simulink library "srx_platform"  (Simulink 8.2)
settings: Solver=ode1  StartTime=0.0  StopTime=Inf  FixedStep=0.001  RelTol=1e-3
PostLoadFcn:
  | , if any(exist('dsrtsu_mdlpostloadfcn', 'file') == [2, 3, 6]), try dsrtsu_mdlpostloadfcn('Execute', bdroot); catch fprintf('Error in PostLoadFcn (dsrtsu_mdlpostloadfcn) for model "%s":\n %s\n', bdroot, lasterr); end, end,
libraries: rtican x23, rtiethernetudplib x4, srx_initialize x4, rtiflashlib x2, topr5_adapter x1
(part 4 of 6)

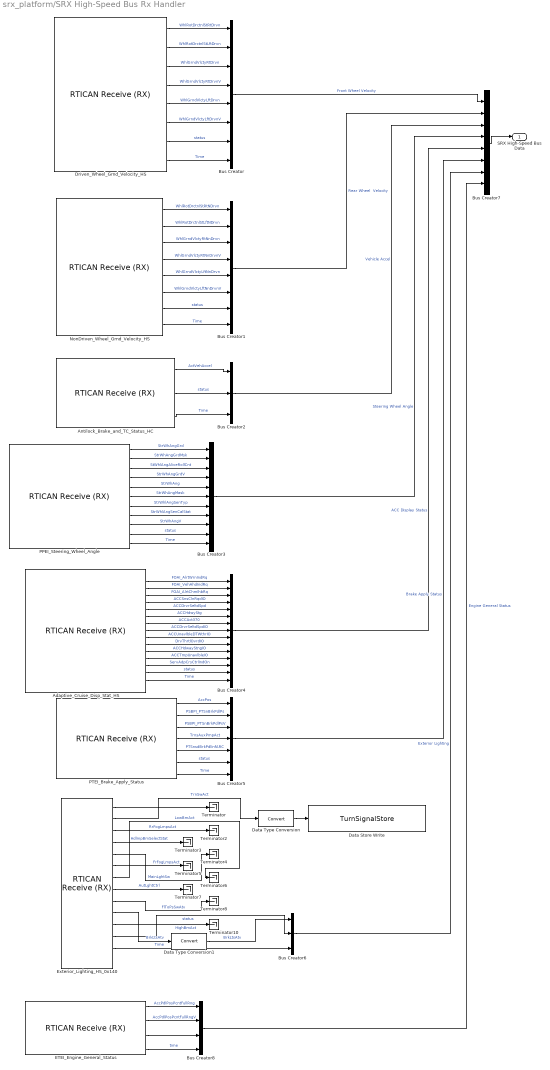
== system srx_platform/SRX High-Speed Bus Rx Handler ==
  Adaptive_Cruise_Disp_Stat_HS : rtican/RTICAN Receive (RX)   Reserved1=[]  Reserved2=[]  Reserved3=[]  Reserved4=[]  SfcnMessage=[]  Msg_Struct=[]  BoardTypeNo=[]  BoardNo=[]  ChannelNo=[]  Parameters=[]  DialogFcn=[]  UnitName=[]  Revision=[]  UnitValues=[]  DSProperties=struct('RTI',struct('Version',uint32(5),'BlockType',struct('isSLSource',uint8(1),'isSLSink',uint8(1),'isHWSource',uint8(0),'isHWSink',uint8(0),'isSetup',uint8(0),'isInline',uint8(1),'isNonInline',uint8(0),'isInterrupt',uint8(0),'isChannelwise',uint8(0)),'IOBoardType','RTICAN','UnitType','MESSAGE','Identifier','RX','DialogType','MSVC','BlockSet','RTICAN','SlaveProcessor','CAN'))  RTIBlockInterface=struct('OutputPortsWidth',int32([1 1 1 1 1 1 1 1 1 1 1 1 1 1 1]),'OutputPortsActive',[1 1 1 1 1 1 1 1 1 1 1 1 1 1 1],'OutputPortsName',{{'FOAI_AlrtWrnIndRq','FOAI_VehAhdIndRq','FOAI_AlrtChmIhbRq','ACCSnsClnRqdIO','ACCDrvrSeltdSpd','ACCHdwyStg','ACCAct370','ACCDrvrSeltdSpdIO','ACCUnavlbleDTWthrIO','DrvThrtlOvrdIO','ACCHdwayStngIO','ACCTmpUnavlbleIO','ServAdpCrsCtrlIndOn',['RX status'],['RX time']}},'OutputPortsDataType',{{'SS_UINT8','SS_UINT8','SS_BOOLEAN','SS_UINT32','SS_DOUBLE','SS_UINT8','SS_BOOLEAN','SS_BOOLEAN','SS_BOOLEAN','SS_BOOLEAN','SS_BOOLEAN','SS_BOOLEAN','SS_BOOLEAN','SS_DOUBLE','SS_DOUBLE'}},'OutputPortsLabel',{{'FOAI_AlrtWrnIndRq','FOAI_VehAhdIndRq','FOAI_AlrtChmIhbRq','ACCSnsClnRqdIO','ACCDrvrSeltdSpd','ACCHdwyStg','ACCAct370','ACCDrvrSeltdSpdIO','ACCUnavlbleDTWthrIO','DrvThrtlOvrdIO','ACCHdwayStngIO','ACCTmpUnavlbleIO','ServAdpCrsCtrlIndOn','',''}},'OutputPortsLabelMode','ON','InputPortsWidth',int32(0),'InputPortsActive',0,'DialogFcn','rtican_message_interface_gui','BlockDisplay',{{'','center'}},'IconTransparency','on','ParameterTunableNames',{{}},'InitLevel',3,'BlockName',struct('Token',{{'Adaptive_Cruise_Disp_Stat_HS'}}),'SampleTime',{{-1}},'TriggerPort',{{'none'}},'EnablePort',{{'none'}})  RTIBlockParameters=struct('BoardTypeNo',{{1,'OFF',[]}},'BoardNo',{{1,'ON',[1 16]}},'ChannelNo',{{1,'ON',[1 2]}},'Parameters',{{struct('DataFileSupport',struct('DataFileSelectedMaster',1,'DataFileSelectedLocal',1,'DataFileName','c:\users\leidos\development\carmaplatform\microautobox\src\data_files\srx_high_speed.dbc|','DataFileDate',{{{['12-Aug-2015 17:10:44']}}},'SelectedFile','..\data_files\srx_high_speed.dbc','InterfaceFcn','rtican_dbc_file_parser'),'Options',struct('StatusSelected',1,'TimeSelected',1,'DeltaTimeSelected',0,'BytePortSelected',0,'MessageLengthSelected',0,'TriggerPort',struct('Selected',0,'TriggerType',0),'UserCoding',struct('Selected',0,'InterfaceFile','UserDecodingFile','FcnName','UserDecodeFcn','InportSelected',0,'InportWidth',1,'OutportSelected',0,'OutportWidth',1),'EnablePortSelected',0,'SignalOnPortnameSelected',1,'UseRXService',1),'Message',struct('MsgOnBlocknameSelected',1,'MsgName','Adaptive_Cruise_Disp_Stat_HS','MsgIdFormat',0,'MsgId',880,'MsgLength',6,'NumSignals',13,'SampleTime',-1,'Signal',struct('SgnName',{'FOAI_AlrtWrnIndRq','FOAI_VehAhdIndRq','FOAI_AlrtChmIhbRq','ACCSnsClnRqdIO','ACCDrvrSeltdSpd','ACCHdwyStg','ACCAct370','ACCDrvrSeltdSpdIO','ACCUnavlbleDTWthrIO','DrvThrtlOvrdIO','ACCHdwayStngIO','ACCTmpUnavlbleIO','ServAdpCrsCtrlIndOn'},'SgnStartBit',{0,4,8,14,16,28,31,41,42,43,44,45,47},'SgnLength',{4,4,1,32,12,3,1,1,1,1,1,1,1},'SgnType',{0,0,0,0,0,0,0,0,0,0,0,0,0},'ModeValue',{-1,-1,-1,-1,-1,-1,-1,-1,-1,-1,-1,-1,-1},'DataType',{0,0,0,0,0,0,0,0,0,0,0,0,0},'ByteLayout',{2,2,2,2,2,2,2,2,2,2,2,2,2},'Factor',{1,1,1,1,0.0625,1,1,1,1,1,1,1,1},'Offset',{0,0,0,0,0,0,0,0,0,0,0,0,0},'SgnComment',{{['Forward Object Alert Indications : Alert Warning Indication Request']},{['Forward Object Alert Indications : Vehicle Ahead Indication Request']},{['Forward Object Alert Indications : Alert Warning Chime Inhibit Request']},{['Adaptive Cruise Control Sensor Cleaning Required Indication On']},{''},{['Adaptive Cruise Control Headway Setting']},{['Adaptive Cruise Control Active']},{['Adaptive Cruise Control Driver Selected Speed Indication On']},{['Adaptive Cruise Unavailable Due To Weather Indication On']},{['Driver Throttle Override Indication On']},{['Adaptive Cruise Control Headway Setting Indication On']},{['Adaptive Cruise Control Temporarily Unavailable Indication On']},{['Service Adaptive Cruise Control Indication On']}},'SgnUnit',{'','','','','km/h','','','','','','','',''},'Min',{0,0,0,0,0,0,0,0,0,0,0,0,0},'Max',{0,0,0,0,0,0,0,0,0,0,0,0,0},'SLDataType',{'SS_UINT8','SS_UINT8','SS_BOOLEAN','SS_UINT32','SS_DOUBLE','SS_UINT8','SS_BOOLEAN','SS_BOOLEAN','SS_BOOLEAN','SS_BOOLEAN','SS_BOOLEAN','SS_BOOLEAN','SS_BOOLEAN'}),'MsgIdNumFormat',0,'MsgComment',{{''}}),'Version',1.2,'general',struct('isFromLib',0)),'OFF',[]}},'GroupId',{{struct('Group',{{'RTICAN'}},'No',1,'Behavior',{{'NAMECHANGE'}},'BlockType',{{'SINK'}},'NameChangeFlag',0),'OFF',[]}},'SFcnRTICANMessage',{{struct('MsgType','RX','SFcnPortType','Scalar','MsgName','Adaptive_Cruise_Disp_Stat_HS','MsgIdFormat','STD','MsgId',880,'MsgLength',6,'NumSignals',13,'SampleTime',-1,'Signal',struct('SgnName',{'FOAI_AlrtWrnIndRq','FOAI_VehAhdIndRq','FOAI_AlrtChmIhbRq','ACCSnsClnRqdIO','ACCDrvrSeltdSpd','ACCHdwyStg','ACCAct370','ACCDrvrSeltdSpdIO','ACCUnavlbleDTWthrIO','DrvThrtlOvrdIO','ACCHdwayStngIO','ACCTmpUnavlbleIO','ServAdpCrsCtrlIndOn'},'SgnStartBit',{0,4,8,14,16,28,31,41,42,43,44,45,47},'SgnLength',{4,4,1,32,12,3,1,1,1,1,1,1,1},'SgnType',{'standard','standard','standard','standard','standard','standard','standard','standard','standard','standard','standard','standard','standard'},'ModeValue',{-1,-1,-1,-1,-1,-1,-1,-1,-1,-1,-1,-1,-1},'DataType',{['unsigned int'],['unsigned int'],['unsigned int'],['unsigned int'],['unsigned int'],['unsigned int'],['unsigned int'],['unsigned int'],['unsigned int'],['unsigned int'],['unsigned int'],['unsigned int'],['unsigned int']},'ByteLayout',{['motorola back.'],['motorola back.'],['motorola back.'],['motorola back.'],['motorola back.'],['motorola back.'],['motorola back.'],['motorola back.'],['motorola back.'],['motorola back.'],['motorola back.'],['motorola back.'],['motorola back.']},'Factor',{1,1,1,1,0.0625,1,1,1,1,1,1,1,1},'Offset',{0,0,0,0,0,0,0,0,0,0,0,0,0},'SLDataType',{'SS_UINT8','SS_UINT8','SS_BOOLEAN','SS_UINT32','SS_DOUBLE','SS_UINT8','SS_BOOLEAN','SS_BOOLEAN','SS_BOOLEAN','SS_BOOLEAN','SS_BOOLEAN','SS_BOOLEAN','SS_BOOLEAN'}),'StatusSelected','yes','TimeSelected','yes','DeltaTimeSelected','no','BytePortSelected','no','MessageLengthSelected','no','TriggerPort',struct('Selected','no','TriggerType',0),'UserCoding',struct('Selected','no','InterfaceFile','UserDecodingFile','FcnName','UserDecodeFcn','InportSelected','no','InportWidth',1,'OutportSelected','no','OutportWidth',1),'EnablePortSelected','no','UseRXService','yes','BoardType','DS1','BoardNo',1,'ControllerNo',1),'OFF',[]}},'TLCFileName',{{'rtican_rx_message','OFF',[]}})  RTISFcnParameters=struct('SFcnRTICANMessage','struct','TLCFileName','char')  RTIBlockParaDefault=struct('BoardTypeNo',4302,'BoardNo',1,'ChannelNo',1,'Parameters',struct('DataFileSupport',struct('DataFileSelectedMaster',0,'DataFileSelectedLocal',0,'DataFileName','','DataFileDate','','SelectedFile',['<no file selected>']),'Options',struct('StatusSelected',1,'TimeSelected',1,'DeltaTimeSelected',1,'BytePortSelected',0,'MessageLengthSelected',0,'TriggerPort',struct('Selected',0,'TriggerType','rising'),'UserCoding',struct('Selected',0,'InterfaceFile','UserDecodingFile','FcnName','UserDecodeFcn','InportSelected',0,'InportWidth',1,'OutportSelected',0,'OutportWidth',1),'EnablePortSelected',0,'SignalOnPortnameSelected',1,'UseRXService',0),'Message',struct('MsgOnBlocknameSelected',0,'MsgName',['RX Message'],'MsgIdFormat',0,'MsgId',100,'MsgLength',8,'NumSignals',1,'SampleTime',-1,'Signal',struct('SgnName',['RX signal'],'SgnStartBit',0,'SgnLength',8,'SgnType',0,'ModeValue',-1,'DataType',0,'SLDataType','SS_DOUBLE','ByteLayout',0,'Factor',1,'Offset',0,'Min',0,'Max',255,'SgnComment',{{}},'SgnUnit',''),'MsgIdNumFormat',0,'MsgComment',{{''}}),'Version',1.2,'general',struct('isFromLib',1)),'GroupId',struct('Group',{{'RTICAN'}},'No',1,'Behavior',{{'NAMECHANGE'}},'BlockType',{{'SINK'}},'NameChangeFlag',0),'SFcnRTICANMessage',struct('MsgType','RX','MsgName',['RX Message'],'MsgIdFormat','STD','MsgId',100,'MsgLength',8,'NumSignals',1,'SampleTime',-1,'Signal',struct('SgnName',['RX signal'],'SgnStartBit',0,'SgnLength',8,'SgnType','standard','ModeValue',-1,'DataType',['unsigned int'],'ByteLayout',['little endian'],'SLDataType','SS_DOUBLE','Factor',1,'Offset',0),'StatusSelected','yes','TimeSelected','yes','DeltaTimeSelected','yes','BytePortSelected','no','MessageLengthSelected','no','EnablePortSelected','no','UserCoding',struct('Selected','no','InterfaceFile','UserDecodingFile','FcnName','UserDecodeFcn','InportSelected','no','InportWidth',1,'OutportSelected','no','OutportWidth',1),'TriggerPort',struct('Selected','no','TriggerType','rising'),'UseRXService','no','BoardType','DS4302','BoardNo',1,'ControllerNo',1,'SFcnPortType','Scalar'),'TLCFileName','rtican_rx_message')
      settings: AttributesFormatString=Group Id: RTICAN1\n
  Antilock_Brake_and_TC_Status_HC : rtican/RTICAN Receive (RX)   Reserved1=[]  Reserved2=[]  Reserved3=[]  Reserved4=[]  SfcnMessage=[]  Msg_Struct=[]  BoardTypeNo=[]  BoardNo=[]  ChannelNo=[]  Parameters=[]  DialogFcn=[]  UnitName=[]  Revision=[]  UnitValues=[]  DSProperties=struct('RTI',struct('Version',uint32(5),'BlockType',struct('isSLSource',uint8(1),'isSLSink',uint8(1),'isHWSource',uint8(0),'isHWSink',uint8(0),'isSetup',uint8(0),'isInline',uint8(1),'isNonInline',uint8(0),'isInterrupt',uint8(0),'isChannelwise',uint8(0)),'IOBoardType','RTICAN','UnitType','MESSAGE','Identifier','RX','DialogType','MSVC','BlockSet','RTICAN','SlaveProcessor','CAN'))  RTIBlockInterface=struct('OutputPortsWidth',int32([1 1 1]),'OutputPortsActive',[1 1 1],'OutputPortsName',{{'ActVehAccel',['RX status'],['RX time']}},'OutputPortsDataType',{{'SS_DOUBLE','SS_DOUBLE','SS_DOUBLE'}},'OutputPortsLabel',{{'ActVehAccel','',''}},'OutputPortsLabelMode','ON','InputPortsWidth',int32(0),'InputPortsActive',0,'DialogFcn','rtican_message_interface_gui','BlockDisplay',{{'','center'}},'IconTransparency','on','ParameterTunableNames',{{}},'InitLevel',3,'BlockName',struct('Token',{{'Antilock_Brake_and_TC_Status_HC'}}),'SampleTime',{{-1}},'TriggerPort',{{'none'}},'EnablePort',{{'none'}})  RTIBlockParameters=struct('BoardTypeNo',{{1,'OFF',[]}},'BoardNo',{{1,'ON',[1 16]}},'ChannelNo',{{1,'ON',[1 2]}},'Parameters',{{struct('DataFileSupport',struct('DataFileSelectedMaster',1,'DataFileSelectedLocal',1,'DataFileName','c:\users\leidos\development\carmaplatform\microautobox\src\data_files\srx_high_speed.dbc|','DataFileDate',{{{['12-Aug-2015 17:10:44']}}},'SelectedFile','..\data_files\srx_high_speed.dbc'),'Options',struct('StatusSelected',1,'TimeSelected',1,'DeltaTimeSelected',0,'BytePortSelected',0,'MessageLengthSelected',0,'TriggerPort',struct('Selected',0,'TriggerType',0),'UserCoding',struct('Selected',0,'InterfaceFile','UserDecodingFile','FcnName','UserDecodeFcn','InportSelected',0,'InportWidth',1,'OutportSelected',0,'OutportWidth',1),'EnablePortSelected',0,'SignalOnPortnameSelected',1,'UseRXService',1),'Message',struct('MsgOnBlocknameSelected',1,'MsgName','Antilock_Brake_and_TC_Status_HC','MsgIdFormat',0,'MsgId',381,'MsgLength',6,'NumSignals',1,'SampleTime',-1,'Signal',struct('SgnName','ActVehAccel','SgnStartBit',0,'SgnLength',12,'SgnType',0,'ModeValue',-1,'DataType',1,'ByteLayout',2,'Factor',0.01,'Offset',0,'SgnComment',{{''}},'SgnUnit','m/s^2','Min',0,'Max',0,'SLDataType','SS_DOUBLE'),'MsgIdNumFormat',0,'MsgComment',{{''}}),'Version',1.2,'general',struct('isFromLib',0)),'OFF',[]}},'GroupId',{{struct('Group',{{'RTICAN'}},'No',1,'Behavior',{{'NAMECHANGE'}},'BlockType',{{'SINK'}},'NameChangeFlag',0),'OFF',[]}},'SFcnRTICANMessage',{{struct('MsgType','RX','SFcnPortType','Scalar','MsgName','Antilock_Brake_and_TC_Status_HC','MsgIdFormat','STD','MsgId',381,'MsgLength',6,'NumSignals',1,'SampleTime',-1,'Signal',struct('SgnName','ActVehAccel','SgnStartBit',0,'SgnLength',12,'SgnType','standard','ModeValue',-1,'DataType',['signed int'],'ByteLayout',['motorola back.'],'Factor',0.01,'Offset',0,'SLDataType','SS_DOUBLE'),'StatusSelected','yes','TimeSelected','yes','DeltaTimeSelected','no','BytePortSelected','no','MessageLengthSelected','no','TriggerPort',struct('Selected','no','TriggerType',0),'UserCoding',struct('Selected','no','InterfaceFile','UserDecodingFile','FcnName','UserDecodeFcn','InportSelected','no','InportWidth',1,'OutportSelected','no','OutportWidth',1),'EnablePortSelected','no','UseRXService','yes','BoardType','DS1','BoardNo',1,'ControllerNo',1),'OFF',[]}},'TLCFileName',{{'rtican_rx_message','OFF',[]}})  RTISFcnParameters=struct('SFcnRTICANMessage','struct','TLCFileName','char')  RTIBlockParaDefault=struct('BoardTypeNo',4302,'BoardNo',1,'ChannelNo',1,'Parameters',struct('DataFileSupport',struct('DataFileSelectedMaster',0,'DataFileSelectedLocal',0,'DataFileName','','DataFileDate','','SelectedFile',['<no file selected>']),'Options',struct('StatusSelected',1,'TimeSelected',1,'DeltaTimeSelected',1,'BytePortSelected',0,'MessageLengthSelected',0,'TriggerPort',struct('Selected',0,'TriggerType','rising'),'UserCoding',struct('Selected',0,'InterfaceFile','UserDecodingFile','FcnName','UserDecodeFcn','InportSelected',0,'InportWidth',1,'OutportSelected',0,'OutportWidth',1),'EnablePortSelected',0,'SignalOnPortnameSelected',1,'UseRXService',0),'Message',struct('MsgOnBlocknameSelected',0,'MsgName',['RX Message'],'MsgIdFormat',0,'MsgId',100,'MsgLength',8,'NumSignals',1,'SampleTime',-1,'Signal',struct('SgnName',['RX signal'],'SgnStartBit',0,'SgnLength',8,'SgnType',0,'ModeValue',-1,'DataType',0,'SLDataType','SS_DOUBLE','ByteLayout',0,'Factor',1,'Offset',0,'Min',0,'Max',255,'SgnComment',{{}},'SgnUnit',''),'MsgIdNumFormat',0,'MsgComment',{{''}}),'Version',1.2,'general',struct('isFromLib',1)),'GroupId',struct('Group',{{'RTICAN'}},'No',1,'Behavior',{{'NAMECHANGE'}},'BlockType',{{'SINK'}},'NameChangeFlag',0),'SFcnRTICANMessage',struct('MsgType','RX','MsgName',['RX Message'],'MsgIdFormat','STD','MsgId',100,'MsgLength',8,'NumSignals',1,'SampleTime',-1,'Signal',struct('SgnName',['RX signal'],'SgnStartBit',0,'SgnLength',8,'SgnType','standard','ModeValue',-1,'DataType',['unsigned int'],'ByteLayout',['little endian'],'SLDataType','SS_DOUBLE','Factor',1,'Offset',0),'StatusSelected','yes','TimeSelected','yes','DeltaTimeSelected','yes','BytePortSelected','no','MessageLengthSelected','no','EnablePortSelected','no','UserCoding',struct('Selected','no','InterfaceFile','UserDecodingFile','FcnName','UserDecodeFcn','InportSelected','no','InportWidth',1,'OutportSelected','no','OutportWidth',1),'TriggerPort',struct('Selected','no','TriggerType','rising'),'UseRXService','no','BoardType','DS4302','BoardNo',1,'ControllerNo',1,'SFcnPortType','Scalar'),'TLCFileName','rtican_rx_message')
      settings: AttributesFormatString=Group Id: RTICAN1\n
  Bus Creator : BusCreator  Inputs=8  NonVirtualBus=on
  Bus Creator1 : BusCreator  Inputs=8
  Bus Creator2 : BusCreator  Inputs=3
  Bus Creator3 : BusCreator  Inputs=11
  Bus Creator4 : BusCreator  Inputs=15
  Bus Creator5 : BusCreator  Inputs=7
  Bus Creator6 : BusCreator  Inputs=3
  Bus Creator7 : BusCreator  Inputs=8
  Bus Creator8 : BusCreator
  Data Store Write : DataStoreWrite  DataStoreName=TurnSignalStore
  Data Type Conversion : DataTypeConversion
  Data Type Conversion1 : DataTypeConversion
  Driven_Wheel_Grnd_Velocity_HS : rtican/RTICAN Receive (RX)   Reserved1=[]  Reserved2=[]  Reserved3=[]  Reserved4=[]  SfcnMessage=[]  Msg_Struct=[]  BoardTypeNo=[]  BoardNo=[]  ChannelNo=[]  Parameters=[]  DialogFcn=[]  UnitName=[]  Revision=[]  UnitValues=[]  DSProperties=struct('RTI',struct('Version',uint32(5),'BlockType',struct('isSLSource',uint8(1),'isSLSink',uint8(1),'isHWSource',uint8(0),'isHWSink',uint8(0),'isSetup',uint8(0),'isInline',uint8(1),'isNonInline',uint8(0),'isInterrupt',uint8(0),'isChannelwise',uint8(0)),'IOBoardType','RTICAN','UnitType','MESSAGE','Identifier','RX','DialogType','MSVC','BlockSet','RTICAN','SlaveProcessor','CAN'))  RTIBlockInterface=struct('OutputPortsWidth',int32([1 1 1 1 1 1 1 1]),'OutputPortsActive',[1 1 1 1 1 1 1 1],'OutputPortsName',{{'WhlRotDrctnlStRtDrvn','WhlRotDrctnlStLftDrvn','WhlGrndVlctyRtDrvn','WhlGrndVlctyRtDrvnV','WhlGrndVlctyLftDrvn','WhlGrndVlctyLftDrvnV',['RX status'],['RX time']}},'OutputPortsDataType',{{'SS_UINT8','SS_UINT8','SS_DOUBLE','SS_BOOLEAN','SS_DOUBLE','SS_BOOLEAN','SS_DOUBLE','SS_DOUBLE'}},'OutputPortsLabel',{{'WhlRotDrctnlStRtDrvn','WhlRotDrctnlStLftDrvn','WhlGrndVlctyRtDrvn','WhlGrndVlctyRtDrvnV','WhlGrndVlctyLftDrvn','WhlGrndVlctyLftDrvnV','',''}},'OutputPortsLabelMode','ON','InputPortsWidth',int32(0),'InputPortsActive',0,'DialogFcn','rtican_message_interface_gui','BlockDisplay',{{'','center'}},'IconTransparency','on','ParameterTunableNames',{{}},'InitLevel',3,'BlockName',struct('Token',{{'Driven_Wheel_Grnd_Velocity_HS'}}),'SampleTime',{{-1}},'TriggerPort',{{'none'}},'EnablePort',{{'none'}})  RTIBlockParameters=struct('BoardTypeNo',{{1,'OFF',[]}},'BoardNo',{{1,'ON',[1 16]}},'ChannelNo',{{1,'ON',[1 2]}},'Parameters',{{struct('DataFileSupport',struct('DataFileSelectedMaster',1,'DataFileSelectedLocal',1,'DataFileName','c:\users\leidos\development\carmaplatform\microautobox\src\data_files\srx_high_speed.dbc|','DataFileDate',{{{['12-Aug-2015 17:10:44']}}},'SelectedFile','..\data_files\srx_high_speed.dbc','InterfaceFcn','rtican_dbc_file_parser'),'Options',struct('StatusSelected',1,'TimeSelected',1,'DeltaTimeSelected',0,'BytePortSelected',0,'MessageLengthSelected',0,'TriggerPort',struct('Selected',0,'TriggerType',0),'UserCoding',struct('Selected',0,'InterfaceFile','UserDecodingFile','FcnName','UserDecodeFcn','InportSelected',0,'InportWidth',1,'OutportSelected',0,'OutportWidth',1),'EnablePortSelected',0,'SignalOnPortnameSelected',1,'UseRXService',1),'Message',struct('MsgOnBlocknameSelected',1,'MsgName','Driven_Wheel_Grnd_Velocity_HS','MsgIdFormat',0,'MsgId',840,'MsgLength',5,'NumSignals',6,'SampleTime',-1,'Signal',struct('SgnName',{'WhlRotDrctnlStRtDrvn','WhlRotDrctnlStLftDrvn','WhlGrndVlctyRtDrvn','WhlGrndVlctyRtDrvnV','WhlGrndVlctyLftDrvn','WhlGrndVlctyLftDrvnV'},'SgnStartBit',{0,3,8,22,24,38},'SgnLength',{3,3,14,1,14,1},'SgnType',{0,0,0,0,0,0},'ModeValue',{-1,-1,-1,-1,-1,-1},'DataType',{0,0,0,0,0,0},'ByteLayout',{2,2,2,2,2,2},'Factor',{1,1,0.03125,1,0.03125,1},'Offset',{0,0,0,0,0,0},'SgnComment',{{''},{''},{''},{''},{''},{''}},'SgnUnit',{'','','km/h','','km/h',''},'Min',{0,0,0,0,0,0},'Max',{0,0,0,0,0,0},'SLDataType',{'SS_UINT8','SS_UINT8','SS_DOUBLE','SS_BOOLEAN','SS_DOUBLE','SS_BOOLEAN'}),'MsgIdNumFormat',0,'MsgComment',{{''}}),'Version',1.2,'general',struct('isFromLib',0)),'OFF',[]}},'GroupId',{{struct('Group',{{'RTICAN'}},'No',1,'Behavior',{{'NAMECHANGE'}},'BlockType',{{'SINK'}},'NameChangeFlag',0),'OFF',[]}},'SFcnRTICANMessage',{{struct('MsgType','RX','SFcnPortType','Scalar','MsgName','Driven_Wheel_Grnd_Velocity_HS','MsgIdFormat','STD','MsgId',840,'MsgLength',5,'NumSignals',6,'SampleTime',-1,'Signal',struct('SgnName',{'WhlRotDrctnlStRtDrvn','WhlRotDrctnlStLftDrvn','WhlGrndVlctyRtDrvn','WhlGrndVlctyRtDrvnV','WhlGrndVlctyLftDrvn','WhlGrndVlctyLftDrvnV'},'SgnStartBit',{0,3,8,22,24,38},'SgnLength',{3,3,14,1,14,1},'SgnType',{'standard','standard','standard','standard','standard','standard'},'ModeValue',{-1,-1,-1,-1,-1,-1},'DataType',{['unsigned int'],['unsigned int'],['unsigned int'],['unsigned int'],['unsigned int'],['unsigned int']},'ByteLayout',{['motorola back.'],['motorola back.'],['motorola back.'],['motorola back.'],['motorola back.'],['motorola back.']},'Factor',{1,1,0.03125,1,0.03125,1},'Offset',{0,0,0,0,0,0},'SLDataType',{'SS_UINT8','SS_UINT8','SS_DOUBLE','SS_BOOLEAN','SS_DOUBLE','SS_BOOLEAN'}),'StatusSelected','yes','TimeSelected','yes','DeltaTimeSelected','no','BytePortSelected','no','MessageLengthSelected','no','TriggerPort',struct('Selected','no','TriggerType',0),'UserCoding',struct('Selected','no','InterfaceFile','UserDecodingFile','FcnName','UserDecodeFcn','InportSelected','no','InportWidth',1,'OutportSelected','no','OutportWidth',1),'EnablePortSelected','no','UseRXService','yes','BoardType','DS1','BoardNo',1,'ControllerNo',1),'OFF',[]}},'TLCFileName',{{'rtican_rx_message','OFF',[]}})  RTISFcnParameters=struct('SFcnRTICANMessage','struct','TLCFileName','char')  RTIBlockParaDefault=struct('BoardTypeNo',4302,'BoardNo',1,'ChannelNo',1,'Parameters',struct('DataFileSupport',struct('DataFileSelectedMaster',0,'DataFileSelectedLocal',0,'DataFileName','','DataFileDate','','SelectedFile',['<no file selected>']),'Options',struct('StatusSelected',1,'TimeSelected',1,'DeltaTimeSelected',1,'BytePortSelected',0,'MessageLengthSelected',0,'TriggerPort',struct('Selected',0,'TriggerType','rising'),'UserCoding',struct('Selected',0,'InterfaceFile','UserDecodingFile','FcnName','UserDecodeFcn','InportSelected',0,'InportWidth',1,'OutportSelected',0,'OutportWidth',1),'EnablePortSelected',0,'SignalOnPortnameSelected',1,'UseRXService',0),'Message',struct('MsgOnBlocknameSelected',0,'MsgName',['RX Message'],'MsgIdFormat',0,'MsgId',100,'MsgLength',8,'NumSignals',1,'SampleTime',-1,'Signal',struct('SgnName',['RX signal'],'SgnStartBit',0,'SgnLength',8,'SgnType',0,'ModeValue',-1,'DataType',0,'SLDataType','SS_DOUBLE','ByteLayout',0,'Factor',1,'Offset',0,'Min',0,'Max',255,'SgnComment',{{}},'SgnUnit',''),'MsgIdNumFormat',0,'MsgComment',{{''}}),'Version',1.2,'general',struct('isFromLib',1)),'GroupId',struct('Group',{{'RTICAN'}},'No',1,'Behavior',{{'NAMECHANGE'}},'BlockType',{{'SINK'}},'NameChangeFlag',0),'SFcnRTICANMessage',struct('MsgType','RX','MsgName',['RX Message'],'MsgIdFormat','STD','MsgId',100,'MsgLength',8,'NumSignals',1,'SampleTime',-1,'Signal',struct('SgnName',['RX signal'],'SgnStartBit',0,'SgnLength',8,'SgnType','standard','ModeValue',-1,'DataType',['unsigned int'],'ByteLayout',['little endian'],'SLDataType','SS_DOUBLE','Factor',1,'Offset',0),'StatusSelected','yes','TimeSelected','yes','DeltaTimeSelected','yes','BytePortSelected','no','MessageLengthSelected','no','EnablePortSelected','no','UserCoding',struct('Selected','no','InterfaceFile','UserDecodingFile','FcnName','UserDecodeFcn','InportSelected','no','InportWidth',1,'OutportSelected','no','OutportWidth',1),'TriggerPort',struct('Selected','no','TriggerType','rising'),'UseRXService','no','BoardType','DS4302','BoardNo',1,'ControllerNo',1,'SFcnPortType','Scalar'),'TLCFileName','rtican_rx_message')
      settings: AttributesFormatString=Group Id: RTICAN1\n
  ETEI_Engine_General_Status : rtican/RTICAN Receive (RX)   Reserved1=[]  Reserved2=[]  Reserved3=[]  Reserved4=[]  SfcnMessage=[]  Msg_Struct=[]  BoardTypeNo=[]  BoardNo=[]  ChannelNo=[]  Parameters=[]  DialogFcn=[]  UnitName=[]  Revision=[]  UnitValues=[]  DSProperties=struct('RTI',struct('Version',uint32(5),'BlockType',struct('isSLSource',uint8(1),'isSLSink',uint8(1),'isHWSource',uint8(0),'isHWSink',uint8(0),'isSetup',uint8(0),'isInline',uint8(1),'isNonInline',uint8(0),'isInterrupt',uint8(0),'isChannelwise',uint8(0)),'IOBoardType','RTICAN','UnitType','MESSAGE','Identifier','RX','DialogType','MSVC','BlockSet','RTICAN','SlaveProcessor','CAN'))  RTIBlockInterface=struct('OutputPortsWidth',int32([1 1 1 1]),'OutputPortsActive',[1 1 1 1],'OutputPortsName',{{'AccPdlPosPcntFullRng','AccPdlPosPcntFullRngV',['RX status'],['RX time']}},'OutputPortsDataType',{{'SS_DOUBLE','SS_BOOLEAN','SS_DOUBLE','SS_DOUBLE'}},'OutputPortsLabel',{{'AccPdlPosPcntFullRng','AccPdlPosPcntFullRngV','',''}},'OutputPortsLabelMode','ON','InputPortsWidth',int32(0),'InputPortsActive',0,'DialogFcn','rtican_message_interface_gui','BlockDisplay',{{'','center'}},'IconTransparency','on','ParameterTunableNames',{{}},'InitLevel',3,'BlockName',struct('Token',{{'ETEI_Engine_General_Status'}}),'SampleTime',{{-1}},'TriggerPort',{{'none'}},'EnablePort',{{'none'}})  RTIBlockParameters=struct('BoardTypeNo',{{1,'OFF',[]}},'BoardNo',{{1,'ON',[1 16]}},'ChannelNo',{{1,'ON',[1 2]}},'Parameters',{{struct('DataFileSupport',struct('DataFileSelectedMaster',1,'DataFileSelectedLocal',1,'DataFileName','c:\users\leidos\development\carmaplatform\microautobox\src\data_files\srx_high_speed.dbc|','DataFileDate',{{{['21-Aug-2015 11:37:23']}}},'SelectedFile','..\data_files\srx_high_speed.dbc'),'Options',struct('StatusSelected',1,'TimeSelected',1,'DeltaTimeSelected',0,'BytePortSelected',0,'MessageLengthSelected',0,'TriggerPort',struct('Selected',0,'TriggerType',0),'UserCoding',struct('Selected',0,'InterfaceFile','UserDecodingFile','FcnName','UserDecodeFcn','InportSelected',0,'InportWidth',1,'OutportSelected',0,'OutportWidth',1),'EnablePortSelected',0,'SignalOnPortnameSelected',1,'UseRXService',0),'Message',struct('MsgOnBlocknameSelected',1,'MsgName','ETEI_Engine_General_Status','MsgIdFormat',0,'MsgId',417,'MsgLength',8,'NumSignals',2,'SampleTime',-1,'Signal',struct('SgnName',{'AccPdlPosPcntFullRng','AccPdlPosPcntFullRngV'},'SgnStartBit',{8,41},'SgnLength',{8,1},'SgnType',{0,0},'ModeValue',{-1,-1},'DataType',{0,0},'ByteLayout',{2,2},'Factor',{0.392157,1},'Offset',{0,0},'SgnComment',{{''},{''}},'SgnUnit',{'%',''},'Min',{0,0},'Max',{0,0},'SLDataType',{'SS_DOUBLE','SS_BOOLEAN'}),'MsgIdNumFormat',0,'MsgComment',{{''}}),'Version',1.2,'general',struct('isFromLib',0)),'OFF',[]}},'GroupId',{{struct('Group',{{'RTICAN'}},'No',1,'Behavior',{{'NAMECHANGE'}},'BlockType',{{'SINK'}},'NameChangeFlag',0),'OFF',[]}},'SFcnRTICANMessage',{{struct('MsgType','RX','SFcnPortType','Scalar','MsgName','ETEI_Engine_General_Status','MsgIdFormat','STD','MsgId',417,'MsgLength',8,'NumSignals',2,'SampleTime',-1,'Signal',struct('SgnName',{'AccPdlPosPcntFullRng','AccPdlPosPcntFullRngV'},'SgnStartBit',{8,41},'SgnLength',{8,1},'SgnType',{'standard','standard'},'ModeValue',{-1,-1},'DataType',{['unsigned int'],['unsigned int']},'ByteLayout',{['motorola back.'],['motorola back.']},'Factor',{0.392157,1},'Offset',{0,0},'SLDataType',{'SS_DOUBLE','SS_BOOLEAN'}),'StatusSelected','yes','TimeSelected','yes','DeltaTimeSelected','no','BytePortSelected','no','MessageLengthSelected','no','TriggerPort',struct('Selected','no','TriggerType',0),'UserCoding',struct('Selected','no','InterfaceFile','UserDecodingFile','FcnName','UserDecodeFcn','InportSelected','no','InportWidth',1,'OutportSelected','no','OutportWidth',1),'EnablePortSelected','no','UseRXService','no','BoardType','DS1','BoardNo',1,'ControllerNo',1),'OFF',[]}},'TLCFileName',{{'rtican_rx_message','OFF',[]}})  RTISFcnParameters=struct('SFcnRTICANMessage','struct','TLCFileName','char')  RTIBlockParaDefault=struct('BoardTypeNo',4302,'BoardNo',1,'ChannelNo',1,'Parameters',struct('DataFileSupport',struct('DataFileSelectedMaster',0,'DataFileSelectedLocal',0,'DataFileName','','DataFileDate','','SelectedFile',['<no file selected>']),'Options',struct('StatusSelected',1,'TimeSelected',1,'DeltaTimeSelected',1,'BytePortSelected',0,'MessageLengthSelected',0,'TriggerPort',struct('Selected',0,'TriggerType','rising'),'UserCoding',struct('Selected',0,'InterfaceFile','UserDecodingFile','FcnName','UserDecodeFcn','InportSelected',0,'InportWidth',1,'OutportSelected',0,'OutportWidth',1),'EnablePortSelected',0,'SignalOnPortnameSelected',1,'UseRXService',0),'Message',struct('MsgOnBlocknameSelected',0,'MsgName',['RX Message'],'MsgIdFormat',0,'MsgId',100,'MsgLength',8,'NumSignals',1,'SampleTime',-1,'Signal',struct('SgnName',['RX signal'],'SgnStartBit',0,'SgnLength',8,'SgnType',0,'ModeValue',-1,'DataType',0,'SLDataType','SS_DOUBLE','ByteLayout',0,'Factor',1,'Offset',0,'Min',0,'Max',255,'SgnComment',{{}},'SgnUnit',''),'MsgIdNumFormat',0,'MsgComment',{{''}}),'Version',1.2,'general',struct('isFromLib',1)),'GroupId',struct('Group',{{'RTICAN'}},'No',1,'Behavior',{{'NAMECHANGE'}},'BlockType',{{'SINK'}},'NameChangeFlag',0),'SFcnRTICANMessage',struct('MsgType','RX','MsgName',['RX Message'],'MsgIdFormat','STD','MsgId',100,'MsgLength',8,'NumSignals',1,'SampleTime',-1,'Signal',struct('SgnName',['RX signal'],'SgnStartBit',0,'SgnLength',8,'SgnType','standard','ModeValue',-1,'DataType',['unsigned int'],'ByteLayout',['little endian'],'SLDataType','SS_DOUBLE','Factor',1,'Offset',0),'StatusSelected','yes','TimeSelected','yes','DeltaTimeSelected','yes','BytePortSelected','no','MessageLengthSelected','no','EnablePortSelected','no','UserCoding',struct('Selected','no','InterfaceFile','UserDecodingFile','FcnName','UserDecodeFcn','InportSelected','no','InportWidth',1,'OutportSelected','no','OutportWidth',1),'TriggerPort',struct('Selected','no','TriggerType','rising'),'UseRXService','no','BoardType','DS4302','BoardNo',1,'ControllerNo',1,'SFcnPortType','Scalar'),'TLCFileName','rtican_rx_message')
      settings: AttributesFormatString=Group Id: RTICAN1\n
  Exterior_Lighting_HS_0x140 : rtican/RTICAN Receive (RX)   Reserved1=[]  Reserved2=[]  Reserved3=[]  Reserved4=[]  SfcnMessage=[]  Msg_Struct=[]  BoardTypeNo=[]  BoardNo=[]  ChannelNo=[]  Parameters=[]  DialogFcn=[]  UnitName=[]  Revision=[]  UnitValues=[]  DSProperties=struct('RTI',struct('Version',uint32(5),'BlockType',struct('isSLSource',uint8(1),'isSLSink',uint8(1),'isHWSource',uint8(0),'isHWSink',uint8(0),'isSetup',uint8(0),'isInline',uint8(1),'isNonInline',uint8(0),'isInterrupt',uint8(0),'isChannelwise',uint8(0)),'IOBoardType','RTICAN','UnitType','MESSAGE','Identifier','RX','DialogType','MSVC','BlockSet','RTICAN','SlaveProcessor','CAN'))  RTIBlockInterface=struct('OutputPortsWidth',int32([1 1 1 1 1 1 1 1 1 1 1 1 1 1]),'OutputPortsActive',[1 1 1 1 1 1 1 1 1 1 1 1 1 1],'OutputPortsName',{{'OtsdAmbtLtLvlStat','TrnSwAct','RrFogLmpsAct','HdlmpBmSelectStat','MainLghtSw','FrFogLmpsAct','LowBmAct','AutLghtCtrl','FlToPsSwAtv','BrkLtsAtv','HighBmAct',['RX status'],['RX time'],['RX delta time']}},'OutputPortsDataType',{{'SS_DOUBLE','SS_DOUBLE','SS_DOUBLE','SS_DOUBLE','SS_DOUBLE','SS_DOUBLE','SS_DOUBLE','SS_DOUBLE','SS_DOUBLE','SS_DOUBLE','SS_DOUBLE','SS_DOUBLE','SS_DOUBLE','SS_DOUBLE'}},'OutputPortsLabel',{{'OtsdAmbtLtLvlStat','TrnSwAct','RrFogLmpsAct','HdlmpBmSelectStat','MainLghtSw','FrFogLmpsAct','LowBmAct','AutLghtCtrl','FlToPsSwAtv','BrkLtsAtv','HighBmAct','','',''}},'OutputPortsLabelMode','ON','InputPortsWidth',int32(0),'InputPortsActive',0,'DialogFcn','rtican_message_interface_gui','BlockDisplay',{{'','center'}},'IconTransparency','on','ParameterTunableNames',{{}},'InitLevel',3,'BlockName',struct('Token',{{'Exterior_Lighting_HS_0x140'}}),'SampleTime',{{-1}},'TriggerPort',{{'none'}},'EnablePort',{{'none'}})  RTIBlockParameters=struct('BoardTypeNo',{{1,'OFF',[]}},'BoardNo',{{1,'ON',[1 16]}},'ChannelNo',{{1,'ON',[1 2]}},'Parameters',{{struct('DataFileSupport',struct('DataFileSelectedMaster',0,'DataFileSelectedLocal',0,'DataFileName',['<no datafile support>|'],'DataFileDate','','SelectedFile',['<no file selected>']),'Options',struct('StatusSelected',1,'TimeSelected',1,'DeltaTimeSelected',1,'BytePortSelected',0,'MessageLengthSelected',0,'TriggerPort',struct('Selected',0,'TriggerType',0),'UserCoding',struct('Selected',0,'InterfaceFile','UserDecodingFile','FcnName','UserDecodeFcn','InportSelected',0,'InportWidth',1,'OutportSelected',0,'OutportWidth',1),'EnablePortSelected',0,'SignalOnPortnameSelected',1,'UseRXService',1),'Message',struct('MsgOnBlocknameSelected',1,'MsgName','Exterior_Lighting_HS_0x140','MsgIdFormat',0,'MsgId',320,'MsgLength',3,'NumSignals',11,'SampleTime',-1,'Signal',struct('SgnName',{'OtsdAmbtLtLvlStat','TrnSwAct','RrFogLmpsAct','HdlmpBmSelectStat','MainLghtSw','FrFogLmpsAct','LowBmAct','AutLghtCtrl','FlToPsSwAtv','BrkLtsAtv','HighBmAct'},'SgnStartBit',{0,2,8,8,11,16,17,20,21,22,23},'SgnLength',{2,2,1,2,2,1,1,1,1,1,1},'SgnType',{0,0,0,0,0,0,0,0,0,0,0},'ModeValue',{-1,-1,-1,-1,-1,-1,-1,-1,-1,-1,-1},'DataType',{0,0,0,0,0,0,0,0,0,0,0},'ByteLayout',{2,2,2,2,2,2,2,2,2,2,2},'Factor',{1,1,1,1,1,1,1,1,1,1,1},'Offset',{0,0,0,0,0,0,0,0,0,0,0},'SgnComment',{{''},{''},{''},{''},{''},{''},{''},{''},{''},{''},{''}},'SgnUnit',{'','','','','','','','','','',''},'Min',{0,0,0,0,0,0,0,0,0,0,0},'Max',{255,255,255,255,255,255,255,255,255,255,255},'SLDataType',{'SS_DOUBLE','SS_DOUBLE','SS_DOUBLE','SS_DOUBLE','SS_DOUBLE','SS_DOUBLE','SS_DOUBLE','SS_DOUBLE','SS_DOUBLE','SS_DOUBLE','SS_DOUBLE'}),'MsgIdNumFormat',1,'MsgComment',{{''}}),'Version',1.2,'general',struct('isFromLib',0)),'OFF',[]}},'GroupId',{{struct('Group',{{'RTICAN'}},'No',1,'Behavior',{{'NAMECHANGE'}},'BlockType',{{'SINK'}},'NameChangeFlag',0),'OFF',[]}},'SFcnRTICANMessage',{{struct('MsgType','RX','SFcnPortType','Scalar','MsgName','Exterior_Lighting_HS_0x140','MsgIdFormat','STD','MsgId',320,'MsgLength',3,'NumSignals',11,'SampleTime',-1,'Signal',struct('SgnName',{'OtsdAmbtLtLvlStat','TrnSwAct','RrFogLmpsAct','HdlmpBmSelectStat','MainLghtSw','FrFogLmpsAct','LowBmAct','AutLghtCtrl','FlToPsSwAtv','BrkLtsAtv','HighBmAct'},'SgnStartBit',{0,2,8,8,11,16,17,20,21,22,23},'SgnLength',{2,2,1,2,2,1,1,1,1,1,1},'SgnType',{'standard','standard','standard','standard','standard','standard','standard','standard','standard','standard','standard'},'ModeValue',{-1,-1,-1,-1,-1,-1,-1,-1,-1,-1,-1},'DataType',{['unsigned int'],['unsigned int'],['unsigned int'],['unsigned int'],['unsigned int'],['unsigned int'],['unsigned int'],['unsigned int'],['unsigned int'],['unsigned int'],['unsigned int']},'ByteLayout',{['motorola back.'],['motorola back.'],['motorola back.'],['motorola back.'],['motorola back.'],['motorola back.'],['motorola back.'],['motorola back.'],['motorola back.'],['motorola back.'],['motorola back.']},'Factor',{1,1,1,1,1,1,1,1,1,1,1},'Offset',{0,0,0,0,0,0,0,0,0,0,0},'SLDataType',{'SS_DOUBLE','SS_DOUBLE','SS_DOUBLE','SS_DOUBLE','SS_DOUBLE','SS_DOUBLE','SS_DOUBLE','SS_DOUBLE','SS_DOUBLE','SS_DOUBLE','SS_DOUBLE'}),'StatusSelected','yes','TimeSelected','yes','DeltaTimeSelected','yes','BytePortSelected','no','MessageLengthSelected','no','TriggerPort',struct('Selected','no','TriggerType',0),'UserCoding',struct('Selected','no','InterfaceFile','UserDecodingFile','FcnName','UserDecodeFcn','InportSelected','no','InportWidth',1,'OutportSelected','no','OutportWidth',1),'EnablePortSelected','no','UseRXService','yes','BoardType','DS1','BoardNo',1,'ControllerNo',1),'OFF',[]}},'TLCFileName',{{'rtican_rx_message','OFF',[]}})  RTISFcnParameters=struct('SFcnRTICANMessage','struct','TLCFileName','char')  RTIBlockParaDefault=struct('BoardTypeNo',4302,'BoardNo',1,'ChannelNo',1,'Parameters',struct('DataFileSupport',struct('DataFileSelectedMaster',0,'DataFileSelectedLocal',0,'DataFileName','','DataFileDate','','SelectedFile',['<no file selected>']),'Options',struct('StatusSelected',1,'TimeSelected',1,'DeltaTimeSelected',1,'BytePortSelected',0,'MessageLengthSelected',0,'TriggerPort',struct('Selected',0,'TriggerType','rising'),'UserCoding',struct('Selected',0,'InterfaceFile','UserDecodingFile','FcnName','UserDecodeFcn','InportSelected',0,'InportWidth',1,'OutportSelected',0,'OutportWidth',1),'EnablePortSelected',0,'SignalOnPortnameSelected',1,'UseRXService',0),'Message',struct('MsgOnBlocknameSelected',0,'MsgName',['RX Message'],'MsgIdFormat',0,'MsgId',100,'MsgLength',8,'NumSignals',1,'SampleTime',-1,'Signal',struct('SgnName',['RX signal'],'SgnStartBit',0,'SgnLength',8,'SgnType',0,'ModeValue',-1,'DataType',0,'SLDataType','SS_DOUBLE','ByteLayout',0,'Factor',1,'Offset',0,'Min',0,'Max',255,'SgnComment',{{}},'SgnUnit',''),'MsgIdNumFormat',0,'MsgComment',{{''}}),'Version',1.2,'general',struct('isFromLib',1)),'GroupId',struct('Group',{{'RTICAN'}},'No',1,'Behavior',{{'NAMECHANGE'}},'BlockType',{{'SINK'}},'NameChangeFlag',0),'SFcnRTICANMessage',struct('MsgType','RX','MsgName',['RX Message'],'MsgIdFormat','STD','MsgId',100,'MsgLength',8,'NumSignals',1,'SampleTime',-1,'Signal',struct('SgnName',['RX signal'],'SgnStartBit',0,'SgnLength',8,'SgnType','standard','ModeValue',-1,'DataType',['unsigned int'],'ByteLayout',['little endian'],'SLDataType','SS_DOUBLE','Factor',1,'Offset',0),'StatusSelected','yes','TimeSelected','yes','DeltaTimeSelected','yes','BytePortSelected','no','MessageLengthSelected','no','EnablePortSelected','no','UserCoding',struct('Selected','no','InterfaceFile','UserDecodingFile','FcnName','UserDecodeFcn','InportSelected','no','InportWidth',1,'OutportSelected','no','OutportWidth',1),'TriggerPort',struct('Selected','no','TriggerType','rising'),'UseRXService','no','BoardType','DS4302','BoardNo',1,'ControllerNo',1,'SFcnPortType','Scalar'),'TLCFileName','rtican_rx_message')
      settings: AttributesFormatString=Group Id: RTICAN1\n
  NonDriven_Wheel_Grnd_Velocity_HS : rtican/RTICAN Receive (RX)   Reserved1=[]  Reserved2=[]  Reserved3=[]  Reserved4=[]  SfcnMessage=[]  Msg_Struct=[]  BoardTypeNo=[]  BoardNo=[]  ChannelNo=[]  Parameters=[]  DialogFcn=[]  UnitName=[]  Revision=[]  UnitValues=[]  DSProperties=struct('RTI',struct('Version',uint32(5),'BlockType',struct('isSLSource',uint8(1),'isSLSink',uint8(1),'isHWSource',uint8(0),'isHWSink',uint8(0),'isSetup',uint8(0),'isInline',uint8(1),'isNonInline',uint8(0),'isInterrupt',uint8(0),'isChannelwise',uint8(0)),'IOBoardType','RTICAN','UnitType','MESSAGE','Identifier','RX','DialogType','MSVC','BlockSet','RTICAN','SlaveProcessor','CAN'))  RTIBlockInterface=struct('OutputPortsWidth',int32([1 1 1 1 1 1 1 1]),'OutputPortsActive',[1 1 1 1 1 1 1 1],'OutputPortsName',{{'WhlRotDrctnlStRtNDrvn','WhlRotDrctnlStLftNDrvn','WhlGrndVlctyRtNnDrvn','WhlGrndVlctyRtNnDrvnV','WhlGrndVlctyLftNnDrvn','WhlGrndVlctyLftNnDrvnV',['RX status'],['RX time']}},'OutputPortsDataType',{{'SS_UINT8','SS_UINT8','SS_DOUBLE','SS_BOOLEAN','SS_DOUBLE','SS_BOOLEAN','SS_DOUBLE','SS_DOUBLE'}},'OutputPortsLabel',{{'WhlRotDrctnlStRtNDrvn','WhlRotDrctnlStLftNDrvn','WhlGrndVlctyRtNnDrvn','WhlGrndVlctyRtNnDrvnV','WhlGrndVlctyLftNnDrvn','WhlGrndVlctyLftNnDrvnV','',''}},'OutputPortsLabelMode','ON','InputPortsWidth',int32(0),'InputPortsActive',0,'DialogFcn','rtican_message_interface_gui','BlockDisplay',{{'','center'}},'IconTransparency','on','ParameterTunableNames',{{}},'InitLevel',3,'BlockName',struct('Token',{{'NonDriven_Wheel_Grnd_Velocity_HS'}}),'SampleTime',{{-1}},'TriggerPort',{{'none'}},'EnablePort',{{'none'}})  RTIBlockParameters=struct('BoardTypeNo',{{1,'OFF',[]}},'BoardNo',{{1,'ON',[1 16]}},'ChannelNo',{{1,'ON',[1 2]}},'Parameters',{{struct('DataFileSupport',struct('DataFileSelectedMaster',1,'DataFileSelectedLocal',1,'DataFileName','c:\users\leidos\development\carmaplatform\microautobox\src\data_files\srx_high_speed.dbc|','DataFileDate',{{{['12-Aug-2015 17:10:44']}}},'SelectedFile','..\data_files\srx_high_speed.dbc','InterfaceFcn','rtican_dbc_file_parser'),'Options',struct('StatusSelected',1,'TimeSelected',1,'DeltaTimeSelected',0,'BytePortSelected',0,'MessageLengthSelected',0,'TriggerPort',struct('Selected',0,'TriggerType',0),'UserCoding',struct('Selected',0,'InterfaceFile','UserDecodingFile','FcnName','UserDecodeFcn','InportSelected',0,'InportWidth',1,'OutportSelected',0,'OutportWidth',1),'EnablePortSelected',0,'SignalOnPortnameSelected',1,'UseRXService',1),'Message',struct('MsgOnBlocknameSelected',1,'MsgName','NonDriven_Wheel_Grnd_Velocity_HS','MsgIdFormat',0,'MsgId',842,'MsgLength',5,'NumSignals',6,'SampleTime',-1,'Signal',struct('SgnName',{'WhlRotDrctnlStRtNDrvn','WhlRotDrctnlStLftNDrvn','WhlGrndVlctyRtNnDrvn','WhlGrndVlctyRtNnDrvnV','WhlGrndVlctyLftNnDrvn','WhlGrndVlctyLftNnDrvnV'},'SgnStartBit',{0,3,8,22,24,38},'SgnLength',{3,3,14,1,14,1},'SgnType',{0,0,0,0,0,0},'ModeValue',{-1,-1,-1,-1,-1,-1},'DataType',{0,0,0,0,0,0},'ByteLayout',{2,2,2,2,2,2},'Factor',{1,1,0.03125,1,0.03125,1},'Offset',{0,0,0,0,0,0},'SgnComment',{{''},{''},{''},{''},{''},{''}},'SgnUnit',{'','','km/h','','km/h',''},'Min',{0,0,0,0,0,0},'Max',{0,0,0,0,0,0},'SLDataType',{'SS_UINT8','SS_UINT8','SS_DOUBLE','SS_BOOLEAN','SS_DOUBLE','SS_BOOLEAN'}),'MsgIdNumFormat',0,'MsgComment',{{''}}),'Version',1.2,'general',struct('isFromLib',0)),'OFF',[]}},'GroupId',{{struct('Group',{{'RTICAN'}},'No',1,'Behavior',{{'NAMECHANGE'}},'BlockType',{{'SINK'}},'NameChangeFlag',0),'OFF',[]}},'SFcnRTICANMessage',{{struct('MsgType','RX','SFcnPortType','Scalar','MsgName','NonDriven_Wheel_Grnd_Velocity_HS','MsgIdFormat','STD','MsgId',842,'MsgLength',5,'NumSignals',6,'SampleTime',-1,'Signal',struct('SgnName',{'WhlRotDrctnlStRtNDrvn','WhlRotDrctnlStLftNDrvn','WhlGrndVlctyRtNnDrvn','WhlGrndVlctyRtNnDrvnV','WhlGrndVlctyLftNnDrvn','WhlGrndVlctyLftNnDrvnV'},'SgnStartBit',{0,3,8,22,24,38},'SgnLength',{3,3,14,1,14,1},'SgnType',{'standard','standard','standard','standard','standard','standard'},'ModeValue',{-1,-1,-1,-1,-1,-1},'DataType',{['unsigned int'],['unsigned int'],['unsigned int'],['unsigned int'],['unsigned int'],['unsigned int']},'ByteLayout',{['motorola back.'],['motorola back.'],['motorola back.'],['motorola back.'],['motorola back.'],['motorola back.']},'Factor',{1,1,0.03125,1,0.03125,1},'Offset',{0,0,0,0,0,0},'SLDataType',{'SS_UINT8','SS_UINT8','SS_DOUBLE','SS_BOOLEAN','SS_DOUBLE','SS_BOOLEAN'}),'StatusSelected','yes','TimeSelected','yes','DeltaTimeSelected','no','BytePortSelected','no','MessageLengthSelected','no','TriggerPort',struct('Selected','no','TriggerType',0),'UserCoding',struct('Selected','no','InterfaceFile','UserDecodingFile','FcnName','UserDecodeFcn','InportSelected','no','InportWidth',1,'OutportSelected','no','OutportWidth',1),'EnablePortSelected','no','UseRXService','yes','BoardType','DS1','BoardNo',1,'ControllerNo',1),'OFF',[]}},'TLCFileName',{{'rtican_rx_message','OFF',[]}})  RTISFcnParameters=struct('SFcnRTICANMessage','struct','TLCFileName','char')  RTIBlockParaDefault=struct('BoardTypeNo',4302,'BoardNo',1,'ChannelNo',1,'Parameters',struct('DataFileSupport',struct('DataFileSelectedMaster',0,'DataFileSelectedLocal',0,'DataFileName','','DataFileDate','','SelectedFile',['<no file selected>']),'Options',struct('StatusSelected',1,'TimeSelected',1,'DeltaTimeSelected',1,'BytePortSelected',0,'MessageLengthSelected',0,'TriggerPort',struct('Selected',0,'TriggerType','rising'),'UserCoding',struct('Selected',0,'InterfaceFile','UserDecodingFile','FcnName','UserDecodeFcn','InportSelected',0,'InportWidth',1,'OutportSelected',0,'OutportWidth',1),'EnablePortSelected',0,'SignalOnPortnameSelected',1,'UseRXService',0),'Message',struct('MsgOnBlocknameSelected',0,'MsgName',['RX Message'],'MsgIdFormat',0,'MsgId',100,'MsgLength',8,'NumSignals',1,'SampleTime',-1,'Signal',struct('SgnName',['RX signal'],'SgnStartBit',0,'SgnLength',8,'SgnType',0,'ModeValue',-1,'DataType',0,'SLDataType','SS_DOUBLE','ByteLayout',0,'Factor',1,'Offset',0,'Min',0,'Max',255,'SgnComment',{{}},'SgnUnit',''),'MsgIdNumFormat',0,'MsgComment',{{''}}),'Version',1.2,'general',struct('isFromLib',1)),'GroupId',struct('Group',{{'RTICAN'}},'No',1,'Behavior',{{'NAMECHANGE'}},'BlockType',{{'SINK'}},'NameChangeFlag',0),'SFcnRTICANMessage',struct('MsgType','RX','MsgName',['RX Message'],'MsgIdFormat','STD','MsgId',100,'MsgLength',8,'NumSignals',1,'SampleTime',-1,'Signal',struct('SgnName',['RX signal'],'SgnStartBit',0,'SgnLength',8,'SgnType','standard','ModeValue',-1,'DataType',['unsigned int'],'ByteLayout',['little endian'],'SLDataType','SS_DOUBLE','Factor',1,'Offset',0),'StatusSelected','yes','TimeSelected','yes','DeltaTimeSelected','yes','BytePortSelected','no','MessageLengthSelected','no','EnablePortSelected','no','UserCoding',struct('Selected','no','InterfaceFile','UserDecodingFile','FcnName','UserDecodeFcn','InportSelected','no','InportWidth',1,'OutportSelected','no','OutportWidth',1),'TriggerPort',struct('Selected','no','TriggerType','rising'),'UseRXService','no','BoardType','DS4302','BoardNo',1,'ControllerNo',1,'SFcnPortType','Scalar'),'TLCFileName','rtican_rx_message')
      settings: AttributesFormatString=Group Id: RTICAN1\n
  PPEI_Steering_Wheel_Angle : rtican/RTICAN Receive (RX)   Reserved1=[]  Reserved2=[]  Reserved3=[]  Reserved4=[]  SfcnMessage=[]  Msg_Struct=[]  BoardTypeNo=[]  BoardNo=[]  ChannelNo=[]  Parameters=[]  DialogFcn=[]  UnitName=[]  Revision=[]  UnitValues=[]  DSProperties=struct('RTI',struct('Version',uint32(5),'BlockType',struct('isSLSource',uint8(1),'isSLSink',uint8(1),'isHWSource',uint8(0),'isHWSink',uint8(0),'isSetup',uint8(0),'isInline',uint8(1),'isNonInline',uint8(0),'isInterrupt',uint8(0),'isChannelwise',uint8(0)),'IOBoardType','RTICAN','UnitType','MESSAGE','Identifier','RX','DialogType','MSVC','BlockSet','RTICAN','SlaveProcessor','CAN'))  RTIBlockInterface=struct('OutputPortsWidth',int32([1 1 1 1 1 1 1 1 1 1 1]),'OutputPortsActive',[1 1 1 1 1 1 1 1 1 1 1],'OutputPortsName',{{'StrWhAngGrd','StrWhAngGrdMsk','StWhlAngAliveRollCnt','StrWhAngGrdV','StrWhAng','StrWhAngMask','StrWhlAngSenTyp','StrWhlAngSenCalStat','StrWhAngV',['RX status'],['RX time']}},'OutputPortsDataType',{{'SS_INT16','SS_BOOLEAN','SS_UINT8','SS_BOOLEAN','SS_DOUBLE','SS_BOOLEAN','SS_UINT8','SS_UINT8','SS_BOOLEAN','SS_DOUBLE','SS_DOUBLE'}},'OutputPortsLabel',{{'StrWhAngGrd','StrWhAngGrdMsk','StWhlAngAliveRollCnt','StrWhAngGrdV','StrWhAng','StrWhAngMask','StrWhlAngSenTyp','StrWhlAngSenCalStat','StrWhAngV','',''}},'OutputPortsLabelMode','ON','InputPortsWidth',int32(0),'InputPortsActive',0,'DialogFcn','rtican_message_interface_gui','BlockDisplay',{{'','center'}},'IconTransparency','on','ParameterTunableNames',{{}},'InitLevel',3,'BlockName',struct('Token',{{'PPEI_Steering_Wheel_Angle'}}),'SampleTime',{{-1}},'TriggerPort',{{'none'}},'EnablePort',{{'none'}})  RTIBlockParameters=struct('BoardTypeNo',{{1,'OFF',[]}},'BoardNo',{{1,'ON',[1 16]}},'ChannelNo',{{1,'ON',[1 2]}},'Parameters',{{struct('DataFileSupport',struct('DataFileSelectedMaster',1,'DataFileSelectedLocal',1,'DataFileName','c:\users\leidos\development\carmaplatform\microautobox\src\data_files\srx_high_speed.dbc|','DataFileDate',{{{['12-Aug-2015 17:10:44']}}},'SelectedFile','..\data_files\srx_high_speed.dbc'),'Options',struct('StatusSelected',1,'TimeSelected',1,'DeltaTimeSelected',0,'BytePortSelected',0,'MessageLengthSelected',0,'TriggerPort',struct('Selected',0,'TriggerType',0),'UserCoding',struct('Selected',0,'InterfaceFile','UserDecodingFile','FcnName','UserDecodeFcn','InportSelected',0,'InportWidth',1,'OutportSelected',0,'OutportWidth',1),'EnablePortSelected',0,'SignalOnPortnameSelected',1,'UseRXService',1),'Message',struct('MsgOnBlocknameSelected',1,'MsgName','PPEI_Steering_Wheel_Angle','MsgIdFormat',0,'MsgId',485,'MsgLength',8,'NumSignals',9,'SampleTime',-1,'Signal',struct('SgnName',{'StrWhAngGrd','StrWhAngGrdMsk','StWhlAngAliveRollCnt','StrWhAngGrdV','StrWhAng','StrWhAngMask','StrWhlAngSenTyp','StrWhlAngSenCalStat','StrWhAngV'},'SgnStartBit',{24,36,37,39,40,58,59,61,63},'SgnLength',{12,1,2,1,16,1,2,2,1},'SgnType',{0,0,0,0,0,0,0,0,0},'ModeValue',{-1,-1,-1,-1,-1,-1,-1,-1,-1},'DataType',{1,0,0,0,1,0,0,0,0},'ByteLayout',{2,2,2,2,2,2,2,2,2},'Factor',{1,1,1,1,0.0625,1,1,1,1},'Offset',{0,0,0,0,0,0,0,0,0},'SgnComment',{{['Steering Wheel Angle Gradient']},{['Steering Wheel Angle Gradient Mask']},{['Steering Wheel Angle Alive Rolling Count']},{['Steering Wheel Angle Gradient Validity']},{['Steering Wheel Angle']},{''},{['Steering Wheel Angle Sensor Type']},{['Steering Wheel Angle Sensor Calibration Status']},{['Steering Wheel Angle Validity']}},'SgnUnit',{'','','','','deg','','','',''},'Min',{0,0,0,0,0,0,0,0,0},'Max',{0,0,0,0,0,0,0,0,0},'SLDataType',{'SS_INT16','SS_BOOLEAN','SS_UINT8','SS_BOOLEAN','SS_DOUBLE','SS_BOOLEAN','SS_UINT8','SS_UINT8','SS_BOOLEAN'}),'MsgIdNumFormat',0,'MsgComment',{{''}}),'Version',1.2,'general',struct('isFromLib',0)),'OFF',[]}},'GroupId',{{struct('Group',{{'RTICAN'}},'No',1,'Behavior',{{'NAMECHANGE'}},'BlockType',{{'SINK'}},'NameChangeFlag',0),'OFF',[]}},'SFcnRTICANMessage',{{struct('MsgType','RX','SFcnPortType','Scalar','MsgName','PPEI_Steering_Wheel_Angle','MsgIdFormat','STD','MsgId',485,'MsgLength',8,'NumSignals',9,'SampleTime',-1,'Signal',struct('SgnName',{'StrWhAngGrd','StrWhAngGrdMsk','StWhlAngAliveRollCnt','StrWhAngGrdV','StrWhAng','StrWhAngMask','StrWhlAngSenTyp','StrWhlAngSenCalStat','StrWhAngV'},'SgnStartBit',{24,36,37,39,40,58,59,61,63},'SgnLength',{12,1,2,1,16,1,2,2,1},'SgnType',{'standard','standard','standard','standard','standard','standard','standard','standard','standard'},'ModeValue',{-1,-1,-1,-1,-1,-1,-1,-1,-1},'DataType',{['signed int'],['unsigned int'],['unsigned int'],['unsigned int'],['signed int'],['unsigned int'],['unsigned int'],['unsigned int'],['unsigned int']},'ByteLayout',{['motorola back.'],['motorola back.'],['motorola back.'],['motorola back.'],['motorola back.'],['motorola back.'],['motorola back.'],['motorola back.'],['motorola back.']},'Factor',{1,1,1,1,0.0625,1,1,1,1},'Offset',{0,0,0,0,0,0,0,0,0},'SLDataType',{'SS_INT16','SS_BOOLEAN','SS_UINT8','SS_BOOLEAN','SS_DOUBLE','SS_BOOLEAN','SS_UINT8','SS_UINT8','SS_BOOLEAN'}),'StatusSelected','yes','TimeSelected','yes','DeltaTimeSelected','no','BytePortSelected','no','MessageLengthSelected','no','TriggerPort',struct('Selected','no','TriggerType',0),'UserCoding',struct('Selected','no','InterfaceFile','UserDecodingFile','FcnName','UserDecodeFcn','InportSelected','no','InportWidth',1,'OutportSelected','no','OutportWidth',1),'EnablePortSelected','no','UseRXService','yes','BoardType','DS1','BoardNo',1,'ControllerNo',1),'OFF',[]}},'TLCFileName',{{'rtican_rx_message','OFF',[]}})  RTISFcnParameters=struct('SFcnRTICANMessage','struct','TLCFileName','char')  RTIBlockParaDefault=struct('BoardTypeNo',4302,'BoardNo',1,'ChannelNo',1,'Parameters',struct('DataFileSupport',struct('DataFileSelectedMaster',0,'DataFileSelectedLocal',0,'DataFileName','','DataFileDate','','SelectedFile',['<no file selected>']),'Options',struct('StatusSelected',1,'TimeSelected',1,'DeltaTimeSelected',1,'BytePortSelected',0,'MessageLengthSelected',0,'TriggerPort',struct('Selected',0,'TriggerType','rising'),'UserCoding',struct('Selected',0,'InterfaceFile','UserDecodingFile','FcnName','UserDecodeFcn','InportSelected',0,'InportWidth',1,'OutportSelected',0,'OutportWidth',1),'EnablePortSelected',0,'SignalOnPortnameSelected',1,'UseRXService',0),'Message',struct('MsgOnBlocknameSelected',0,'MsgName',['RX Message'],'MsgIdFormat',0,'MsgId',100,'MsgLength',8,'NumSignals',1,'SampleTime',-1,'Signal',struct('SgnName',['RX signal'],'SgnStartBit',0,'SgnLength',8,'SgnType',0,'ModeValue',-1,'DataType',0,'SLDataType','SS_DOUBLE','ByteLayout',0,'Factor',1,'Offset',0,'Min',0,'Max',255,'SgnComment',{{}},'SgnUnit',''),'MsgIdNumFormat',0,'MsgComment',{{''}}),'Version',1.2,'general',struct('isFromLib',1)),'GroupId',struct('Group',{{'RTICAN'}},'No',1,'Behavior',{{'NAMECHANGE'}},'BlockType',{{'SINK'}},'NameChangeFlag',0),'SFcnRTICANMessage',struct('MsgType','RX','MsgName',['RX Message'],'MsgIdFormat','STD','MsgId',100,'MsgLength',8,'NumSignals',1,'SampleTime',-1,'Signal',struct('SgnName',['RX signal'],'SgnStartBit',0,'SgnLength',8,'SgnType','standard','ModeValue',-1,'DataType',['unsigned int'],'ByteLayout',['little endian'],'SLDataType','SS_DOUBLE','Factor',1,'Offset',0),'StatusSelected','yes','TimeSelected','yes','DeltaTimeSelected','yes','BytePortSelected','no','MessageLengthSelected','no','EnablePortSelected','no','UserCoding',struct('Selected','no','InterfaceFile','UserDecodingFile','FcnName','UserDecodeFcn','InportSelected','no','InportWidth',1,'OutportSelected','no','OutportWidth',1),'TriggerPort',struct('Selected','no','TriggerType','rising'),'UseRXService','no','BoardType','DS4302','BoardNo',1,'ControllerNo',1,'SFcnPortType','Scalar'),'TLCFileName','rtican_rx_message')
      settings: AttributesFormatString=Group Id: RTICAN1\n
  PTEI_Brake_Apply_Status : rtican/RTICAN Receive (RX)   Reserved1=[]  Reserved2=[]  Reserved3=[]  Reserved4=[]  SfcnMessage=[]  Msg_Struct=[]  BoardTypeNo=[]  BoardNo=[]  ChannelNo=[]  Parameters=[]  DialogFcn=[]  UnitName=[]  Revision=[]  UnitValues=[]  DSProperties=struct('RTI',struct('Version',uint32(5),'BlockType',struct('isSLSource',uint8(1),'isSLSink',uint8(1),'isHWSource',uint8(0),'isHWSink',uint8(0),'isSetup',uint8(0),'isInline',uint8(1),'isNonInline',uint8(0),'isInterrupt',uint8(0),'isChannelwise',uint8(0)),'IOBoardType','RTICAN','UnitType','MESSAGE','Identifier','RX','DialogType','MSVC','BlockSet','RTICAN','SlaveProcessor','CAN'))  RTIBlockInterface=struct('OutputPortsWidth',int32([1 1 1 1 1 1 1]),'OutputPortsActive',[1 1 1 1 1 1 1],'OutputPortsName',{{'AccPos','PSBPI_PTSnBrkPdlPs','PSBPI_PTSnBrkPdlPsV','TrnsAuxPmpAct','PTSnsdBrkPdlInfARC',['RX status'],['RX time']}},'OutputPortsDataType',{{'SS_DOUBLE','SS_DOUBLE','SS_BOOLEAN','SS_BOOLEAN','SS_UINT8','SS_DOUBLE','SS_DOUBLE'}},'OutputPortsLabel',{{'AccPos','PSBPI_PTSnBrkPdlPs','PSBPI_PTSnBrkPdlPsV','TrnsAuxPmpAct','PTSnsdBrkPdlInfARC','',''}},'OutputPortsLabelMode','ON','InputPortsWidth',int32(0),'InputPortsActive',0,'DialogFcn','rtican_message_interface_gui','BlockDisplay',{{'','center'}},'IconTransparency','on','ParameterTunableNames',{{}},'InitLevel',3,'BlockName',struct('Token',{{'PTEI_Brake_Apply_Status'}}),'SampleTime',{{-1}},'TriggerPort',{{'none'}},'EnablePort',{{'none'}})  RTIBlockParameters=struct('BoardTypeNo',{{1,'OFF',[]}},'BoardNo',{{1,'ON',[1 16]}},'ChannelNo',{{1,'ON',[1 2]}},'Parameters',{{struct('DataFileSupport',struct('DataFileSelectedMaster',1,'DataFileSelectedLocal',1,'DataFileName','c:\users\leidos\development\carmaplatform\microautobox\src\data_files\srx_high_speed.dbc|','DataFileDate',{{{['12-Aug-2015 17:10:44']}}},'SelectedFile','..\data_files\srx_high_speed.dbc'),'Options',struct('StatusSelected',1,'TimeSelected',1,'DeltaTimeSelected',0,'BytePortSelected',0,'MessageLengthSelected',0,'TriggerPort',struct('Selected',0,'TriggerType',0),'UserCoding',struct('Selected',0,'InterfaceFile','UserDecodingFile','FcnName','UserDecodeFcn','InportSelected',0,'InportWidth',1,'OutportSelected',0,'OutportWidth',1),'EnablePortSelected',0,'SignalOnPortnameSelected',1,'UseRXService',1),'Message',struct('MsgOnBlocknameSelected',1,'MsgName','PTEI_Brake_Apply_Status','MsgIdFormat',0,'MsgId',190,'MsgLength',5,'NumSignals',5,'SampleTime',-1,'Signal',struct('SgnName',{'AccPos','PSBPI_PTSnBrkPdlPs','PSBPI_PTSnBrkPdlPsV','TrnsAuxPmpAct','PTSnsdBrkPdlInfARC'},'SgnStartBit',{16,24,32,33,34},'SgnLength',{8,8,1,1,2},'SgnType',{0,0,0,0,0},'ModeValue',{-1,-1,-1,-1,-1},'DataType',{0,0,0,0,0},'ByteLayout',{2,2,2,2,2},'Factor',{0.392157,0.392157,1,1,1},'Offset',{0,0,0,0,0},'SgnComment',{{['Accelerator Effective Position']},{['Powertrain Sensed Brake Pedal Position']},{['Powertrain Sensed Brake Pedal Position Validity']},{['Transmission Auxiliary Pump Active']},{['Powertrain Sensed Brake Pedal Information Alive Rolling Count']}},'SgnUnit',{'%','%','','',''},'Min',{0,0,0,0,0},'Max',{0,0,0,0,0},'SLDataType',{'SS_DOUBLE','SS_DOUBLE','SS_BOOLEAN','SS_BOOLEAN','SS_UINT8'}),'MsgIdNumFormat',0,'MsgComment',{{''}}),'Version',1.2,'general',struct('isFromLib',0)),'OFF',[]}},'GroupId',{{struct('Group',{{'RTICAN'}},'No',1,'Behavior',{{'NAMECHANGE'}},'BlockType',{{'SINK'}},'NameChangeFlag',0),'OFF',[]}},'SFcnRTICANMessage',{{struct('MsgType','RX','SFcnPortType','Scalar','MsgName','PTEI_Brake_Apply_Status','MsgIdFormat','STD','MsgId',190,'MsgLength',5,'NumSignals',5,'SampleTime',-1,'Signal',struct('SgnName',{'AccPos','PSBPI_PTSnBrkPdlPs','PSBPI_PTSnBrkPdlPsV','TrnsAuxPmpAct','PTSnsdBrkPdlInfARC'},'SgnStartBit',{16,24,32,33,34},'SgnLength',{8,8,1,1,2},'SgnType',{'standard','standard','standard','standard','standard'},'ModeValue',{-1,-1,-1,-1,-1},'DataType',{['unsigned int'],['unsigned int'],['unsigned int'],['unsigned int'],['unsigned int']},'ByteLayout',{['motorola back.'],['motorola back.'],['motorola back.'],['motorola back.'],['motorola back.']},'Factor',{0.392157,0.392157,1,1,1},'Offset',{0,0,0,0,0},'SLDataType',{'SS_DOUBLE','SS_DOUBLE','SS_BOOLEAN','SS_BOOLEAN','SS_UINT8'}),'StatusSelected','yes','TimeSelected','yes','DeltaTimeSelected','no','BytePortSelected','no','MessageLengthSelected','no','TriggerPort',struct('Selected','no','TriggerType',0),'UserCoding',struct('Selected','no','InterfaceFile','UserDecodingFile','FcnName','UserDecodeFcn','InportSelected','no','InportWidth',1,'OutportSelected','no','OutportWidth',1),'EnablePortSelected','no','UseRXService','yes','BoardType','DS1','BoardNo',1,'ControllerNo',1),'OFF',[]}},'TLCFileName',{{'rtican_rx_message','OFF',[]}})  RTISFcnParameters=struct('SFcnRTICANMessage','struct','TLCFileName','char')  RTIBlockParaDefault=struct('BoardTypeNo',4302,'BoardNo',1,'ChannelNo',1,'Parameters',struct('DataFileSupport',struct('DataFileSelectedMaster',0,'DataFileSelectedLocal',0,'DataFileName','','DataFileDate','','SelectedFile',['<no file selected>']),'Options',struct('StatusSelected',1,'TimeSelected',1,'DeltaTimeSelected',1,'BytePortSelected',0,'MessageLengthSelected',0,'TriggerPort',struct('Selected',0,'TriggerType','rising'),'UserCoding',struct('Selected',0,'InterfaceFile','UserDecodingFile','FcnName','UserDecodeFcn','InportSelected',0,'InportWidth',1,'OutportSelected',0,'OutportWidth',1),'EnablePortSelected',0,'SignalOnPortnameSelected',1,'UseRXService',0),'Message',struct('MsgOnBlocknameSelected',0,'MsgName',['RX Message'],'MsgIdFormat',0,'MsgId',100,'MsgLength',8,'NumSignals',1,'SampleTime',-1,'Signal',struct('SgnName',['RX signal'],'SgnStartBit',0,'SgnLength',8,'SgnType',0,'ModeValue',-1,'DataType',0,'SLDataType','SS_DOUBLE','ByteLayout',0,'Factor',1,'Offset',0,'Min',0,'Max',255,'SgnComment',{{}},'SgnUnit',''),'MsgIdNumFormat',0,'MsgComment',{{''}}),'Version',1.2,'general',struct('isFromLib',1)),'GroupId',struct('Group',{{'RTICAN'}},'No',1,'Behavior',{{'NAMECHANGE'}},'BlockType',{{'SINK'}},'NameChangeFlag',0),'SFcnRTICANMessage',struct('MsgType','RX','MsgName',['RX Message'],'MsgIdFormat','STD','MsgId',100,'MsgLength',8,'NumSignals',1,'SampleTime',-1,'Signal',struct('SgnName',['RX signal'],'SgnStartBit',0,'SgnLength',8,'SgnType','standard','ModeValue',-1,'DataType',['unsigned int'],'ByteLayout',['little endian'],'SLDataType','SS_DOUBLE','Factor',1,'Offset',0),'StatusSelected','yes','TimeSelected','yes','DeltaTimeSelected','yes','BytePortSelected','no','MessageLengthSelected','no','EnablePortSelected','no','UserCoding',struct('Selected','no','InterfaceFile','UserDecodingFile','FcnName','UserDecodeFcn','InportSelected','no','InportWidth',1,'OutportSelected','no','OutportWidth',1),'TriggerPort',struct('Selected','no','TriggerType','rising'),'UseRXService','no','BoardType','DS4302','BoardNo',1,'ControllerNo',1,'SFcnPortType','Scalar'),'TLCFileName','rtican_rx_message')
      settings: AttributesFormatString=Group Id: RTICAN1\n
  Terminator{,2..8,10} (9 alike) : Terminator
  SRX High-Speed Bus Data : Outport
  wires:
  Driven_Wheel_Grnd_Velocity_HS/7 -> Bus Creator/7  "status"
  Driven_Wheel_Grnd_Velocity_HS/8 -> Bus Creator/8  "Time"
  NonDriven_Wheel_Grnd_Velocity_HS/6 -> Bus Creator1/6  "WhlGrndVlctyLftNnDrvnV"
  NonDriven_Wheel_Grnd_Velocity_HS/7 -> Bus Creator1/7  "status"
  NonDriven_Wheel_Grnd_Velocity_HS/8 -> Bus Creator1/8  "Time"
  Antilock_Brake_and_TC_Status_HC/2 -> Bus Creator2/2  "status"
  Antilock_Brake_and_TC_Status_HC/1 -> Bus Creator2/1  "ActVehAccel"
  Antilock_Brake_and_TC_Status_HC/3 -> Bus Creator2/3  "Time"
  Bus Creator/1 -> Bus Creator7/1  "Front Wheel Velocity"
  Bus Creator1/1 -> Bus Creator7/2  "Rear Wheel  Velocity"
  Bus Creator2/1 -> Bus Creator7/3  "Vehicle Accel"
  Bus Creator3/1 -> Bus Creator7/4  "Steering Wheel Angle"
  Exterior_Lighting_HS_0x140/12 -> Bus Creator6/2  "status"
  Exterior_Lighting_HS_0x140/13 -> Bus Creator6/3  "Time"
  Bus Creator6/1 -> Bus Creator7/7  "Exterior Lighting"
  Bus Creator5/1 -> Bus Creator7/6  "Brake Apply Status"
  Bus Creator7/1 -> SRX High-Speed Bus Data/1
  Driven_Wheel_Grnd_Velocity_HS/1 -> Bus Creator/1  "WhlRotDrctnlStRtDrvn"
  Driven_Wheel_Grnd_Velocity_HS/2 -> Bus Creator/2  "WhlRotDrctnlStLftDrvn"
  Driven_Wheel_Grnd_Velocity_HS/4 -> Bus Creator/4  "WhlGrndVlctyRtDrvnV"
  Driven_Wheel_Grnd_Velocity_HS/5 -> Bus Creator/5  "WhlGrndVlctyLftDrvn"
  Driven_Wheel_Grnd_Velocity_HS/6 -> Bus Creator/6  "WhlGrndVlctyLftDrvnV"
  Driven_Wheel_Grnd_Velocity_HS/3 -> Bus Creator/3  "WhlGrndVlctyRtDrvn"
  NonDriven_Wheel_Grnd_Velocity_HS/4 -> Bus Creator1/4  "WhlGrndVlctyRtNnDrvnV"
  NonDriven_Wheel_Grnd_Velocity_HS/3 -> Bus Creator1/3  "WhlGrndVlctyRtNnDrvn"
  NonDriven_Wheel_Grnd_Velocity_HS/5 -> Bus Creator1/5  "WhlGrndVlctyLftNnDrvn"
  NonDriven_Wheel_Grnd_Velocity_HS/2 -> Bus Creator1/2  "WhlRotDrctnlStLftNDrvn"
  NonDriven_Wheel_Grnd_Velocity_HS/1 -> Bus Creator1/1  "WhlRotDrctnlStRtNDrvn"
  PPEI_Steering_Wheel_Angle/6 -> Bus Creator3/6  "StrWhAngMask"
  PPEI_Steering_Wheel_Angle/8 -> Bus Creator3/8  "StrWhlAngSenCalStat"
  PPEI_Steering_Wheel_Angle/11 -> Bus Creator3/11  "Time"
  PPEI_Steering_Wheel_Angle/10 -> Bus Creator3/10  "status"
  PPEI_Steering_Wheel_Angle/2 -> Bus Creator3/2  "StrWhAngGrdMsk"
  PPEI_Steering_Wheel_Angle/7 -> Bus Creator3/7  "StrWhlAngSenTyp"
  PPEI_Steering_Wheel_Angle/1 -> Bus Creator3/1  "StrWhAngGrd"
  PPEI_Steering_Wheel_Angle/5 -> Bus Creator3/5  "StrWhAng"
  PPEI_Steering_Wheel_Angle/3 -> Bus Creator3/3  "StWhlAngAliveRollCnt"
  PPEI_Steering_Wheel_Angle/4 -> Bus Creator3/4  "StrWhAngGrdV"
  PPEI_Steering_Wheel_Angle/9 -> Bus Creator3/9  "StrWhAngV"
  Adaptive_Cruise_Disp_Stat_HS/14 -> Bus Creator4/14  "status"
  Adaptive_Cruise_Disp_Stat_HS/9 -> Bus Creator4/9  "ACCUnavlbleDTWthrIO"
  Adaptive_Cruise_Disp_Stat_HS/1 -> Bus Creator4/1  "FOAI_AlrtWrnIndRq"
  Adaptive_Cruise_Disp_Stat_HS/6 -> Bus Creator4/6  "ACCHdwyStg"
  Adaptive_Cruise_Disp_Stat_HS/11 -> Bus Creator4/11  "ACCHdwayStngIO"
  Adaptive_Cruise_Disp_Stat_HS/12 -> Bus Creator4/12  "ACCTmpUnavlbleIO"
  Adaptive_Cruise_Disp_Stat_HS/4 -> Bus Creator4/4  "ACCSnsClnRqdIO"
  Adaptive_Cruise_Disp_Stat_HS/8 -> Bus Creator4/8  "ACCDrvrSeltdSpdIO"
  Adaptive_Cruise_Disp_Stat_HS/5 -> Bus Creator4/5  "ACCDrvrSeltdSpd"
  Adaptive_Cruise_Disp_Stat_HS/7 -> Bus Creator4/7  "ACCAct370"
  Adaptive_Cruise_Disp_Stat_HS/3 -> Bus Creator4/3  "FOAI_AlrtChmIhbRq"
  Adaptive_Cruise_Disp_Stat_HS/13 -> Bus Creator4/13  "ServAdpCrsCtrlIndOn"
  Adaptive_Cruise_Disp_Stat_HS/2 -> Bus Creator4/2  "FOAI_VehAhdIndRq"
  Adaptive_Cruise_Disp_Stat_HS/10 -> Bus Creator4/10  "DrvThrtlOvrdIO"
  Adaptive_Cruise_Disp_Stat_HS/15 -> Bus Creator4/15  "Time"
  PTEI_Brake_Apply_Status/1 -> Bus Creator5/1  "AccPos"
  PTEI_Brake_Apply_Status/5 -> Bus Creator5/5  "PTSnsdBrkPdlInfARC"
  PTEI_Brake_Apply_Status/6 -> Bus Creator5/6  "status"
  PTEI_Brake_Apply_Status/4 -> Bus Creator5/4  "TrnsAuxPmpAct"
  PTEI_Brake_Apply_Status/7 -> Bus Creator5/7  "Time"
  PTEI_Brake_Apply_Status/3 -> Bus Creator5/3  "PSBPI_PTSnBrkPdlPsV"
  PTEI_Brake_Apply_Status/2 -> Bus Creator5/2  "PSBPI_PTSnBrkPdlPs"
  Bus Creator4/1 -> Bus Creator7/5  "ACC Display Status"
  Bus Creator8/1 -> Bus Creator7/8  "Engine General Status"
  ETEI_Engine_General_Status/3 -> Bus Creator8/3
  ETEI_Engine_General_Status/4 -> Bus Creator8/4  "time"
  ETEI_Engine_General_Status/1 -> Bus Creator8/1  "AccPdlPosPcntFullRng"
  ETEI_Engine_General_Status/2 -> Bus Creator8/2  "AccPdlPosPcntFullRngV"
  Exterior_Lighting_HS_0x140/11 -> Terminator10/1  "HighBmAct"
  Exterior_Lighting_HS_0x140/10 -> Data Type Conversion1/1  "BrkLtsAtv"
  Exterior_Lighting_HS_0x140/3 -> Terminator2/1  "RrFogLmpsAct"
  Exterior_Lighting_HS_0x140/2 -> Data Type Conversion/1  "TrnSwAct"
  Exterior_Lighting_HS_0x140/5 -> Terminator4/1  "MainLghtSw"
  Exterior_Lighting_HS_0x140/6 -> Terminator5/1  "FrFogLmpsAct"
  Exterior_Lighting_HS_0x140/4 -> Terminator3/1  "HdlmpBmSelectStat"
  Exterior_Lighting_HS_0x140/8 -> Terminator7/1  "AutLghtCtrl"
  Exterior_Lighting_HS_0x140/7 -> Terminator6/1  "LowBmAct"
  Exterior_Lighting_HS_0x140/9 -> Terminator8/1  "FlToPsSwAtv"
  Data Type Conversion/1 -> Data Store Write/1
  Exterior_Lighting_HS_0x140/1 -> Terminator/1
  Data Type Conversion1/1 -> Bus Creator6/1  "BrkLtsAtv"
